simulink model "cylinder"  (R2019b)
settings: Solver=VariableStepAuto  StartTime=0.0  StopTime=5  RelTol=1e-3
undefined symbols (not defined in the file): gamma, L, p_A0, p_B0, R, S_A, S_B, T, V_0A, V_0B, x0
settings Model: Creator=artof  LastModifiedBy=artof

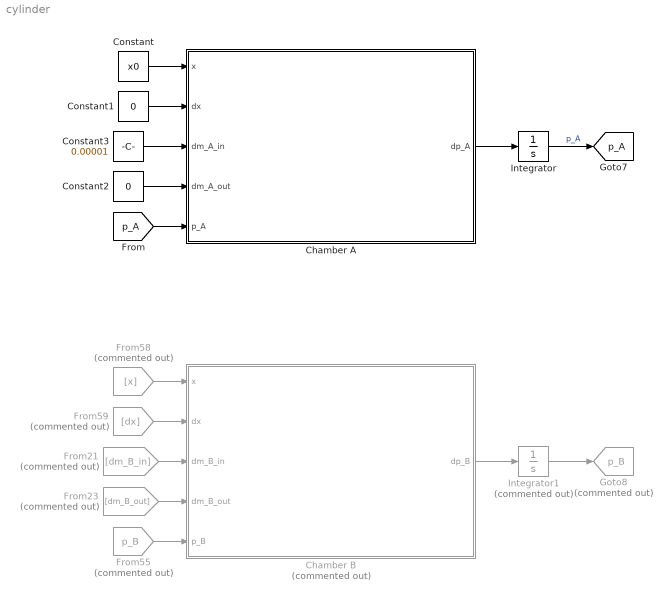
== system cylinder ==
  Chamber A : Subsystem
  Chamber B : Subsystem  Commented=on
  Constant : Constant  Value=x0
  Constant1 : Constant  Value=0
  Constant2 : Constant  Value=0
  Constant3 : Constant  Value=0.00001
  From21 : From  Commented=on  GotoTag=dm_B_in  TagVisibility=global
  From23 : From  Commented=on  GotoTag=dm_B_out  TagVisibility=global
  From55 : From  Commented=on  GotoTag=p_B  TagVisibility=global
  From58 : From  Commented=on  GotoTag=x  TagVisibility=global
  From59 : From  Commented=on  GotoTag=dx  TagVisibility=global
  Goto8 : Goto  Commented=on  GotoTag=p_B  TagVisibility=global
  Integrator : Integrator  InitialCondition=p_A0
  Integrator1 : Integrator  Commented=on  InitialCondition=p_B0
  tag scope: p_A=global
  wires:
  Constant1/1 -> Chamber A/2(dx)
  From23/1 -> Chamber B/4(dm_B_out)
  Constant2/1 -> Chamber A/4(dm_A_out)
  Integrator1/1 -> Goto8/1
  Constant/1 -> Chamber A/1(x)
  Constant3/1 -> Chamber A/3(dm_A_in)
  From58/1 -> Chamber B/1(x)
  From55/1 -> Chamber B/5(p_B)
  Chamber A/1(dp_A) -> Integrator/1
  Chamber B/1(dp_B) -> Integrator1/1
  From21/1 -> Chamber B/3(dm_B_in)
  From59/1 -> Chamber B/2(dx)
  [p_A] -> Chamber A/5(p_A)
  Integrator/1 -> [p_A]  "p_A"

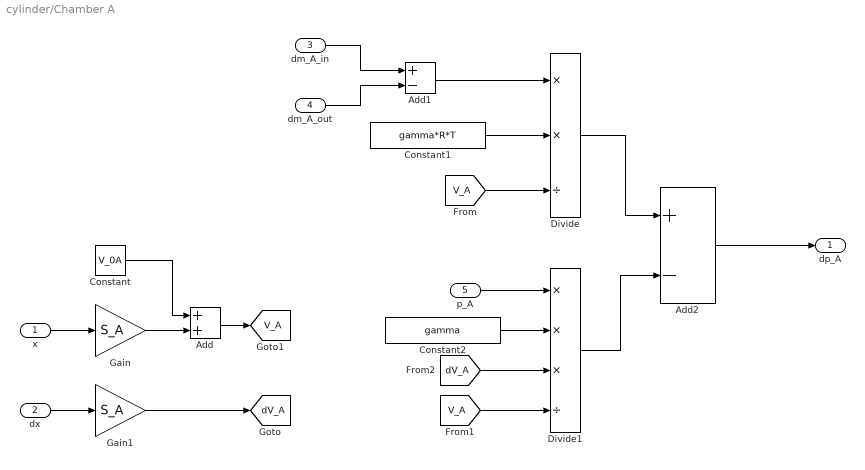
== system cylinder/Chamber A ==
  x : Inport
  dx : Inport  Port=2
  dm_A_in : Inport  Port=3
  dm_A_out : Inport  Port=4
  p_A : Inport  Port=5
  Add : Sum
  Add1 : Sum  Inputs=+-
  Add2 : Sum  Inputs=+-
  Constant : Constant  Value=V_0A
  Constant1 : Constant  Value=gamma*R*T
  Constant2 : Constant  Value=gamma
  Divide : Product  Inputs=**/
  Divide1 : Product  Inputs=***/
  Gain : Gain  Gain=S_A
  Gain1 : Gain  Gain=S_A
  dp_A : Outport
  tag scope: V_A=global, dV_A=global
  wires:
  x/1 -> Gain/1
  Gain/1 -> Add/2
  Constant/1 -> Add/1
  dx/1 -> Gain1/1
  Gain1/1 -> [dV_A]
  Add/1 -> [V_A]
  dm_A_out/1 -> Add1/2
  dm_A_in/1 -> Add1/1
  Add1/1 -> Divide/1
  Constant1/1 -> Divide/2
  [V_A] -> Divide/3
  Divide/1 -> Add2/1
  p_A/1 -> Divide1/1
  Constant2/1 -> Divide1/2
  [V_A] -> Divide1/4
  [dV_A] -> Divide1/3
  Divide1/1 -> Add2/2
  Add2/1 -> dp_A/1

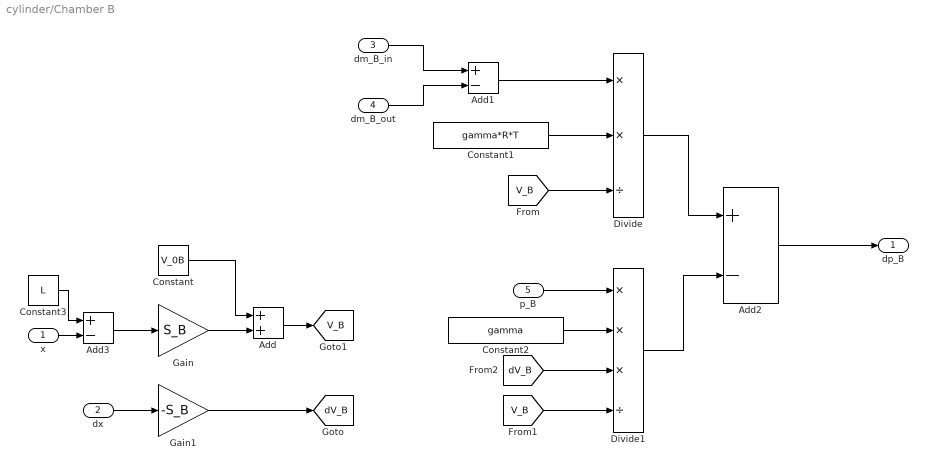
== system cylinder/Chamber B ==
  x : Inport
  dx : Inport  Port=2
  dm_B_in : Inport  Port=3
  dm_B_out : Inport  Port=4
  p_B : Inport  Port=5
  Add : Sum
  Add1 : Sum  Inputs=+-
  Add2 : Sum  Inputs=+-
  Add3 : Sum  Inputs=+-
  Constant : Constant  Value=V_0B
  Constant1 : Constant  Value=gamma*R*T
  Constant2 : Constant  Value=gamma
  Constant3 : Constant  Value=L
  Divide : Product  Inputs=**/
  Divide1 : Product  Inputs=***/
  Gain : Gain  Gain=S_B
  Gain1 : Gain  Gain=-S_B
  dp_B : Outport
  tag scope: V_B=global, dV_B=global
  wires:
  Add2/1 -> dp_B/1
  Divide1/1 -> Add2/2
  [dV_B] -> Divide1/3
  [V_B] -> Divide1/4
  Constant2/1 -> Divide1/2
  p_B/1 -> Divide1/1
  Divide/1 -> Add2/1
  [V_B] -> Divide/3
  Constant1/1 -> Divide/2
  Add1/1 -> Divide/1
  dm_B_in/1 -> Add1/1
  dm_B_out/1 -> Add1/2
  Add/1 -> [V_B]
  Gain1/1 -> [dV_B]
  dx/1 -> Gain1/1
  Constant/1 -> Add/1
  Gain/1 -> Add/2
  x/1 -> Add3/2
  Add3/1 -> Gain/1
  Constant3/1 -> Add3/1
